simulink model "lab0_sim_deg"  (R2022b)
settings: Solver=ode45  StartTime=0.0  StopTime=45  RelTol=1e-3
values from neighbouring files (symbols this model uses):
  degs2rpm = 60/360    (= 0.166666666667)    [load_params_inertial_case.m]    (also in parameters 2.mat; parameters.mat)
  der =     [parameters 2.mat]    (also in parameters.mat)
  pid =     [parameters 2.mat]    (also in parameters.mat)
  rpm2degs = 360/60    (= 6)    [load_params_inertial_case.m]    (also in parameters 2.mat; parameters.mat)
  sens =     [parameters 2.mat]    (also in parameters.mat)
libraries: simulink x3
settings Model: Creator=emanuelevitetta  LastModifiedBy=david

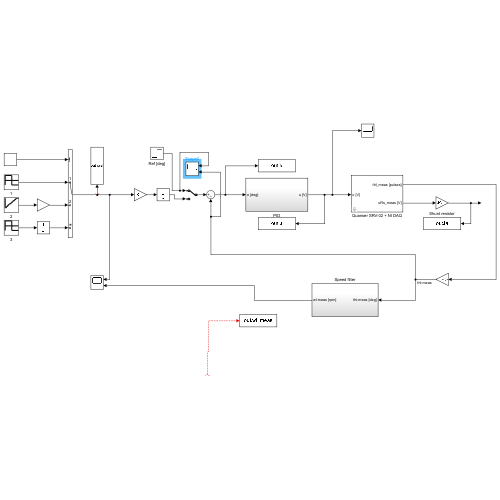
[thumbnail: Simulink's stored preview of the top-level diagram]
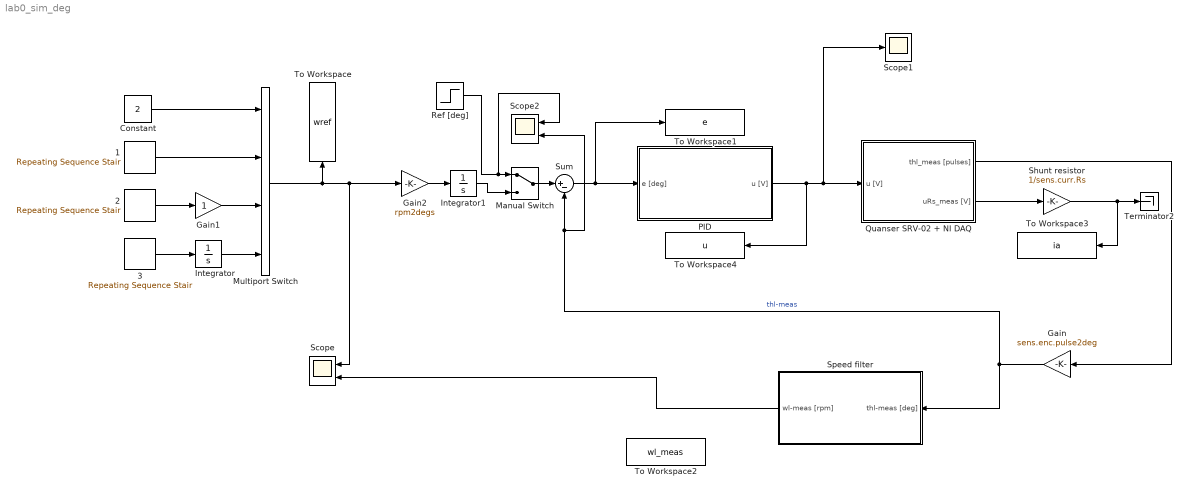
== system lab0_sim_deg ==
  1 : simulink/Sources/Repeating Sequence Stair  OutValues=[250 -250].'  tsamp=1  OutMin=[]  OutMax=[]  OutDataTypeStr=double  OutputDataTypeScalingMode=double  OutDataType=fixdt(0,8)  ConRadixGroup=Best Precision: Vector-wise  OutScaling=2^-12
  2 : simulink/Sources/Repeating Sequence Stair  OutValues=[50 100 150 200 250 300 350 400 450 450].'  tsamp=5  OutMin=[]  OutMax=[]  OutDataTypeStr=double  OutputDataTypeScalingMode=double  OutDataType=fixdt(0,8)  ConRadixGroup=Best Precision: Vector-wise  OutScaling=2^-12
  3 : simulink/Sources/Repeating Sequence Stair  OutValues=[450 -450].'  tsamp=1  OutMin=[]  OutMax=[]  OutDataTypeStr=double  OutputDataTypeScalingMode=double  OutDataType=fixdt(0,8)  ConRadixGroup=Best Precision: Vector-wise  OutScaling=2^-12
  Constant : Constant  Value=2
  Gain : Gain  Gain=sens.enc.pulse2deg
  Gain1 : Gain
  Gain2 : Gain  Gain=rpm2degs
  Integrator : Integrator
  Integrator1 : Integrator
  Manual Switch : ManualSwitch
  Multiport Switch : MultiPortSwitch  SaturateOnIntegerOverflow=off  InputSameDT=off
  PID : Subsystem
  Quanser SRV-02 + NI DAQ : Subsystem  mask(Quanser SRV-02 (with inertial load) + NI DAQ){Ts=0.001, fricType=Coulomb + viscous}
      mask prompts: Ts "NI DAQ Sample Time:"; fricType "Friction model"
      mask help: Quanser SRV-02 (with inertial load) + NI DAQ model.
      mask init:
      | %%  Sensors data
      | 
      | %   shunt resistor
      | sens.curr.Rs = 0.5;                         %   resistance [Ohm]   
      | sens.curr.uRs_std = 0.01;                   %   voltage noise standard dev [V]                           
      | sens.curr.uRs_var = sens.curr.uRs_std^2;	%   voltage noise variance [V^2]
      | 
      | %   Hewlett-Packard HEDS-5540#A06 optical encoder
      | sens.enc.ppr = 500*4;                       %   pulses per rotation
      | sens.enc.pulse2deg = 360/sens.enc.ppr;      %   [pulses] -> [deg]
      | sens.enc.pulse2rad = 2*pi/sens.enc.ppr;     %   [pulses] -> [rad]
      | sens.enc.deg2pulse = sens.enc.ppr/360;      %   [deg] -> [pulses]
      | sens.enc.rad2pulse = sens.enc.ppr/2/pi;     %   [rad] -> [pulses]
      | 
      | 
      | %%  Data acquisition board (daq) data
      | 
      | %   NI PCI-6221 DAC data
      | daq.dac.bits = 16;                                  %   resolution (bits)
      | daq.dac.fs   = 10;                                  %   full scale 
      | daq.dac.q    = 2*daq.dac.fs/(2^daq.dac.bits-1);     %	quantization
      | 
      | %   NI PCI-6221 ADC data
      | daq.adc.bits = 16;                                  %   resolution (bits)
      | daq.adc.fs   = 10;                                  %   full scale (as set in SLDRT Analog Input block)
      | daq.adc.q    = 2*daq.adc.fs/(2^daq.adc.bits-1);     %   quantization
      mask Help:
      | Riccardo Antonello (antonello@dei.unipd.it)
      | 
      | April 24, 2020
      | 
      | Dept. of Information Engineering, University of Padova
      mask TypeOptions fricType: Coulomb + viscous | Karnopp
  Ref [deg] : Step
  Scope : Scope  NumInputPorts=2
  Scope1 : Scope
  Scope2 : Scope  NumInputPorts=2
  Shunt resistor : Gain  Gain=1/sens.curr.Rs
  Speed filter : Subsystem
  Sum : Sum  Inputs=|+-
  Terminator2 : Terminator
  To Workspace : ToWorkspace  VariableName=wref  SaveFormat=Timeseries  SampleTime=-1
  To Workspace1 : ToWorkspace  VariableName=e  SaveFormat=Timeseries  SampleTime=-1
  To Workspace2 : ToWorkspace  VariableName=wl_meas  SaveFormat=Timeseries  SampleTime=-1
  To Workspace3 : ToWorkspace  VariableName=ia  SaveFormat=Timeseries  SampleTime=-1
  To Workspace4 : ToWorkspace  VariableName=u  SaveFormat=Timeseries  SampleTime=-1
  wires:
  PID/1(u [V]) -> To Workspace4/1, Scope1/1, Quanser SRV-02 + NI DAQ/1(u [V])
  Quanser SRV-02 + NI DAQ/1(thl_meas [pulses]) -> Gain/1
  Gain/1 -> Scope2/2, Sum/2, Speed filter/1(thl-meas [deg])  "thl-meas"
  Quanser SRV-02 + NI DAQ/2(uRs_meas [V]) -> Shunt resistor/1
  Sum/1 -> To Workspace1/1, PID/1(e [deg])
  Shunt resistor/1 -> To Workspace3/1, Terminator2/1
  ? -> To Workspace2/1
  3/1 -> Integrator/1
  1/1 -> Multiport Switch/2
  Integrator/1 -> Multiport Switch/4
  Constant/1 -> Multiport Switch/1
  Gain1/1 -> Multiport Switch/3
  2/1 -> Gain1/1
  Speed filter/1(wl-meas [rpm]) -> Scope/2
  Gain2/1 -> Integrator1/1
  Multiport Switch/1 -> Scope/1, Gain2/1, To Workspace/1
  Integrator1/1 -> Manual Switch/2
  Manual Switch/1 -> Sum/1
  Ref [deg]/1 -> Scope2/1, Manual Switch/1

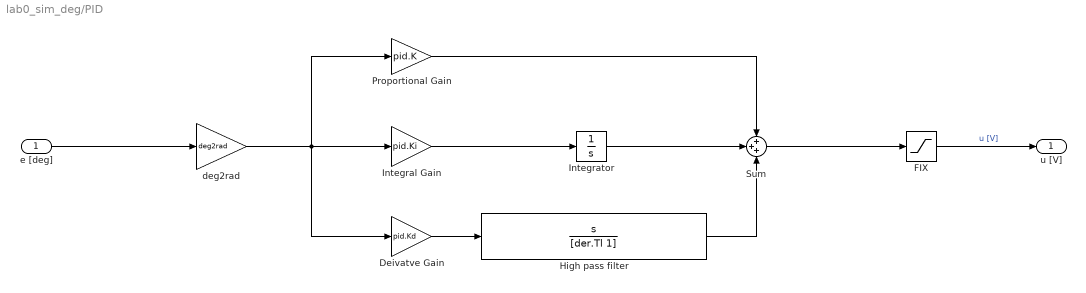
== system lab0_sim_deg/PID ==
  e [deg] : Inport
  Deivatve Gain : Gain  Gain=pid.Kd
  "FIX " : Saturate  UpperLimit=10  LowerLimit=-10
  High pass filter : TransferFcn  Numerator=[1 0]  Denominator=[der.Tl 1]
  Integral Gain : Gain  Gain=pid.Ki
  Integrator : Integrator
  Proportional Gain : Gain  Gain=pid.K
  Sum : Sum  Inputs=+++
  deg2rad : Gain  Gain=deg2rad
  u [V] : Outport
  wires:
  Deivatve Gain/1 -> High pass filter/1
  e [deg]/1 -> deg2rad/1
  Integrator/1 -> Sum/2
  "FIX "/1 -> u [V]/1  "u [V]"
  deg2rad/1 -> Deivatve Gain/1, Proportional Gain/1, Integral Gain/1
  High pass filter/1 -> Sum/3
  Integral Gain/1 -> Integrator/1
  Proportional Gain/1 -> Sum/1
  Sum/1 -> "FIX "/1

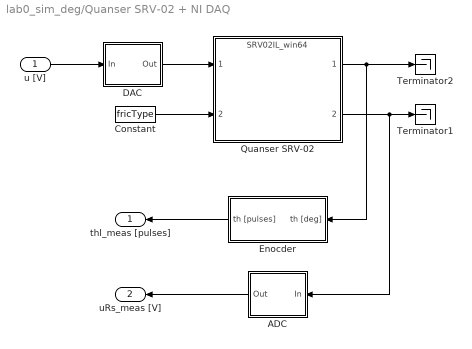
== system lab0_sim_deg/Quanser SRV-02 + NI DAQ ==
  u [V] : Inport
  ADC : Subsystem
  Constant : Constant  Value=fricType
  DAC : Subsystem
  Enocder : Subsystem
  Quanser SRV-02 : ModelReference  ModelNameDialog=SRV02IL_win64.slxp  ModelReferenceVersion=1.44  CopyOfModelProtected=on
  Terminator1 : Terminator
  Terminator2 : Terminator
  thl_meas [pulses] : Outport
  uRs_meas [V] : Outport  Port=2
  wires:
  Enocder/1(th [pulses]) -> thl_meas [pulses]/1
  ADC/1(Out) -> uRs_meas [V]/1
  DAC/1(Out) -> Quanser SRV-02/1
  Quanser SRV-02/2 -> ADC/1(In), Terminator1/1
  u [V]/1 -> DAC/1(In)
  Quanser SRV-02/1 -> Enocder/1(th [deg]), Terminator2/1
  Constant/1 -> Quanser SRV-02/2

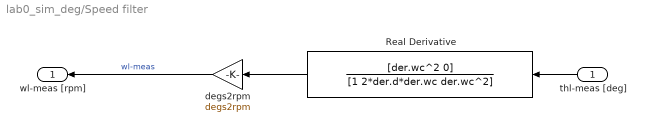
== system lab0_sim_deg/Speed filter ==
  thl-meas [deg] : Inport
  Real Derivative : TransferFcn  Numerator=[der.wc^2 0]  Denominator=[1 2*der.d*der.wc der.wc^2]
  degs2rpm : Gain  Gain=degs2rpm
  wl-meas [rpm] : Outport
  wires:
  thl-meas [deg]/1 -> Real Derivative/1
  degs2rpm/1 -> wl-meas [rpm]/1  "wl-meas"
  Real Derivative/1 -> degs2rpm/1

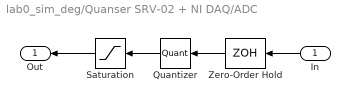
== system lab0_sim_deg/Quanser SRV-02 + NI DAQ/ADC ==
  In : Inport
  Quantizer : Quantizer  QuantizationInterval=daq.adc.q
  Saturation : Saturate  UpperLimit=daq.adc.fs  LowerLimit=-daq.adc.fs
  Zero-Order Hold : ZeroOrderHold  SampleTime=Ts
  Out : Outport
  wires:
  Saturation/1 -> Out/1
  In/1 -> Zero-Order Hold/1
  Quantizer/1 -> Saturation/1
  Zero-Order Hold/1 -> Quantizer/1

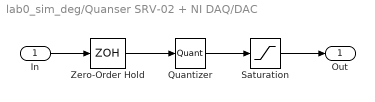
== system lab0_sim_deg/Quanser SRV-02 + NI DAQ/DAC ==
  In : Inport
  Quantizer : Quantizer  QuantizationInterval=daq.dac.q
  Saturation : Saturate  UpperLimit=daq.dac.fs  LowerLimit=-daq.dac.fs
  Zero-Order Hold : ZeroOrderHold  SampleTime=Ts
  Out : Outport
  wires:
  Quantizer/1 -> Saturation/1
  In/1 -> Zero-Order Hold/1
  Zero-Order Hold/1 -> Quantizer/1
  Saturation/1 -> Out/1

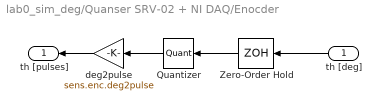
== system lab0_sim_deg/Quanser SRV-02 + NI DAQ/Enocder ==
  th [deg] : Inport
  Quantizer : Quantizer  QuantizationInterval=sens.enc.pulse2deg
  Zero-Order Hold : ZeroOrderHold  SampleTime=Ts
  deg2pulse : Gain  Gain=sens.enc.deg2pulse
  th [pulses] : Outport
  wires:
  Quantizer/1 -> deg2pulse/1
  th [deg]/1 -> Zero-Order Hold/1
  Zero-Order Hold/1 -> Quantizer/1
  deg2pulse/1 -> th [pulses]/1
